simulink model "PMSG"  (Simulink 8.1)
settings: Solver=ode45  StartTime=0.0  StopTime=10  RelTol=1e-3
libraries: simulink x1
settings Model: Creator=korichi  LastModifiedBy=apple
settings SolverCC: ZeroCrossAlgorithm=Adaptive
settings OptimizationCC: InitFltsAndDblsToZero=on
settings DebuggingCC: StrictBusMsg=Warning

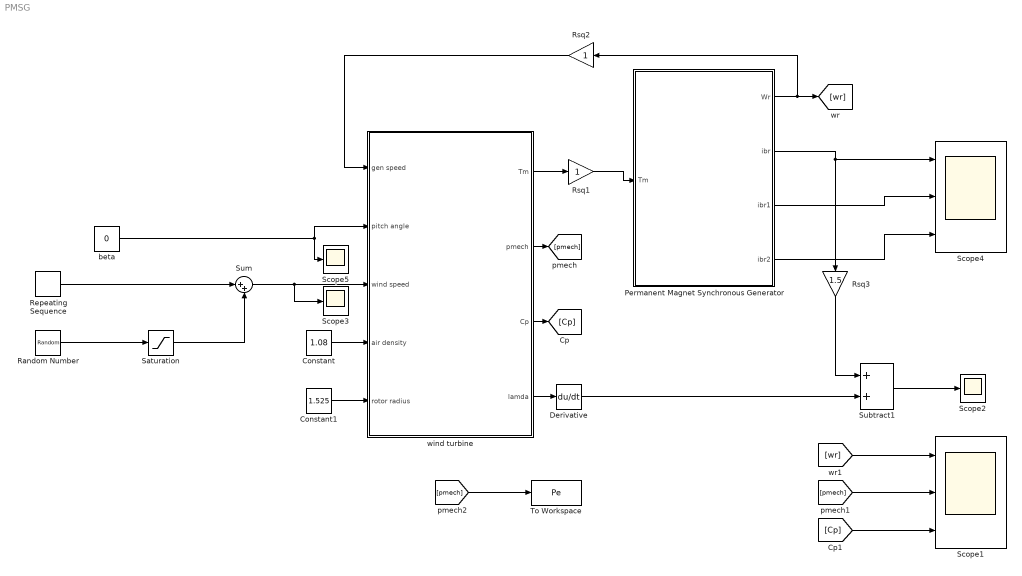
== system PMSG ==
  Constant : Constant  Value=1.08
  Constant1 : Constant  Value=1.525
  Derivative : Derivative
  Permanent Magnet Synchronous Generator : Subsystem
  Random Number : RandomNumber  Seed=20  SampleTime=0
  Repeating Sequence : simulink/Sources/Repeating Sequence  rep_seq_t=[0 2]  rep_seq_y=[0 2]
  Rsq1 : Gain
  Rsq2 : Gain
  Rsq3 : Gain  Gain=1.5
  Saturation : Saturate  UpperLimit=12  LowerLimit=5
  Scope1 : Scope  NumInputPorts=3
      settings: YMin=200~0~-0.3  YMax=650~10000~0.3  SaveName=TeW2  MaxDataPoints=100000000
  Scope2 : Scope
      settings: TimeRange=10  YMin=-9  YMax=9  SaveName=TeW  MaxDataPoints=100000000  SampleInput=on
  Scope3 : Scope
      settings: TimeRange=10  YMin=5  YMax=20  SaveName=TeW3  MaxDataPoints=100000000  SampleInput=on
  Scope4 : Scope  NumInputPorts=3
      settings: YMin=-0.7~-0.7~-0.7  YMax=0.7~0.7~0.7  SaveName=TeW1  MaxDataPoints=100000000
  Scope5 : Scope
      settings: TimeRange=10  YMin=0  YMax=55  SaveName=TeW4  MaxDataPoints=100000000  SampleInput=on
  Subtract1 : Sum
  Sum : Sum  Inputs=|++
  To Workspace : ToWorkspace  VariableName=Pe  SampleTime=-1  SaveFormat=Structure
  beta : Constant  Value=0
  wind turbine : Subsystem
  wires:
  Constant/1 -> wind turbine/4(air density)
  Constant1/1 -> wind turbine/5(rotor radius)
  wind turbine/1(Tm) -> Rsq1/1
  Sum/1 -> wind turbine/3(wind speed), Scope3/1
  Rsq2/1 -> wind turbine/1(gen speed)
  Rsq1/1 -> Permanent Magnet Synchronous Generator/1(Tm)
  wind turbine/3(Cp) -> [Cp]
  wind turbine/2(pmech) -> [pmech]
  [Cp] -> Scope1/3
  [pmech] -> Scope1/2
  [wr] -> Scope1/1
  Permanent Magnet Synchronous Generator/2(ibr) -> Scope4/1, Rsq3/1
  Rsq3/1 -> Subtract1/1
  wind turbine/4(lamda) -> Derivative/1
  Derivative/1 -> Subtract1/2
  Permanent Magnet Synchronous Generator/1(Wr) -> Rsq2/1, [wr]
  Saturation/1 -> Sum/2
  Subtract1/1 -> Scope2/1
  [pmech] -> To Workspace/1
  Permanent Magnet Synchronous Generator/3(ibr1) -> Scope4/2
  Permanent Magnet Synchronous Generator/4(ibr2) -> Scope4/3
  beta/1 -> wind turbine/2(pitch angle), Scope5/1
  Random Number/1 -> Saturation/1
  Repeating Sequence/1 -> Sum/1

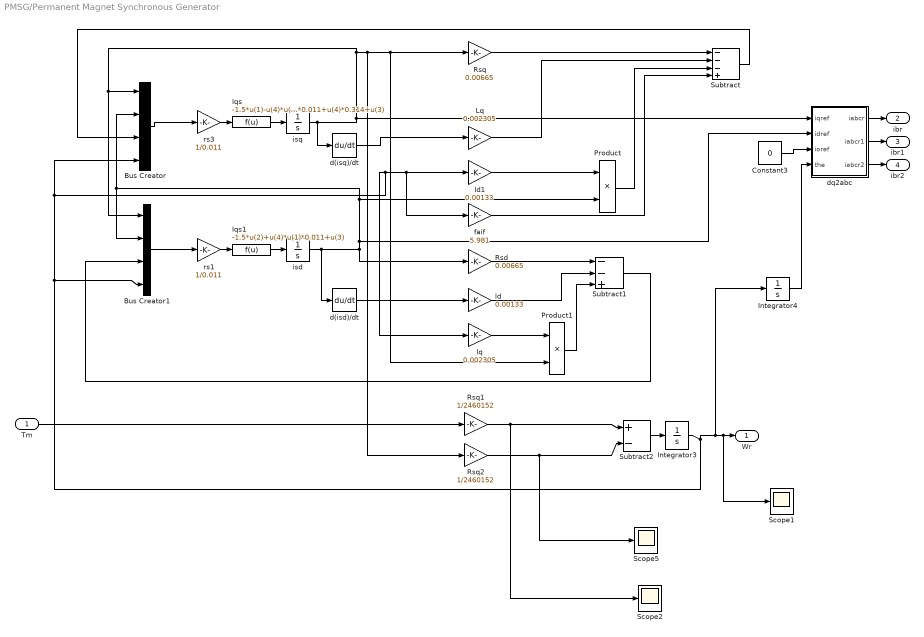
== system PMSG/Permanent Magnet Synchronous Generator ==
  Tm : Inport
  Bus Creator : BusCreator
  Bus Creator1 : BusCreator
  Constant3 : Constant  Value=0
  Integrator3 : Integrator  InitialCondition=1  IgnoreLimit=on
  Integrator4 : Integrator
  Iqs : Fcn  Expr=-1.5*u(1)-u(4)*u(2)*0.011+u(4)*0.314+u(3)
  Iqs1 : Fcn  Expr=-1.5*u(2)+u(4)*u(1)*0.011+u(3)
  Lq : Gain  Gain=0.002305
  Product : Product  RndMeth=Zero
  Product1 : Product  RndMeth=Zero
  Rsd : Gain  Gain=0.00665
  Rsq : Gain  Gain=0.00665  SampleTime=0.00665
  Rsq1 : Gain  Gain=1/2460152
  Rsq2 : Gain  Gain=1/2460152
  Scope1 : Scope
      settings: TimeRange=10  YMin=150  YMax=425  SaveName=TeW6  MaxDataPoints=100000000  SampleInput=on
  Scope2 : Scope
      settings: TimeRange=10  YMin=46.6  YMax=48.3  SaveName=TeW7  MaxDataPoints=100000000  SampleInput=on
  Scope5 : Scope
      settings: TimeRange=10  YMin=0.0035  YMax=0.00625  SaveName=TeW5  MaxDataPoints=100000000  SampleInput=on
  Subtract : Sum  Inputs=---+
  Subtract1 : Sum  Inputs=--+
  Subtract2 : Sum  Inputs=+-
  d(isd)/dt : Derivative
  d(isq)/dt : Derivative
  dq2abc : Subsystem
  faif : Gain  Gain=5.981
  isd : Integrator
  isq : Integrator
  ld : Gain  Gain=0.00133
  ld1 : Gain  Gain=0.00133
  lq : Gain  Gain=0.002305
  rs1 : Gain  Gain=1/0.011
  rs3 : Gain  Gain=1/0.011
  Wr : Outport
  ibr : Outport  Port=2
  ibr1 : Outport  Port=3
  ibr2 : Outport  Port=4
  wires:
  Rsq/1 -> Subtract/1
  Iqs/1 -> isq/1
  rs3/1 -> Iqs/1
  Bus Creator/1 -> rs3/1
  Rsq1/1 -> Scope2/1, Subtract2/1
  Rsq2/1 -> Scope5/1, Subtract2/2
  Subtract2/1 -> Integrator3/1
  Iqs1/1 -> isd/1
  rs1/1 -> Iqs1/1
  Bus Creator1/1 -> rs1/1
  Constant3/1 -> dq2abc/3(ioref)
  dq2abc/1(iabcr) -> ibr/1
  isq/1 -> Bus Creator/1, Bus Creator1/1, Rsq/1, Product1/2, Rsq2/1, dq2abc/1(iqref), d(isq)/dt/1
  isd/1 -> Bus Creator1/2, Bus Creator/2, Product/2, dq2abc/2(idref), Rsd/1, d(isd)/dt/1
  Lq/1 -> Subtract/2
  ld1/1 -> Product/1
  Product/1 -> Subtract/3
  faif/1 -> Subtract/4
  Rsd/1 -> Subtract1/1
  ld/1 -> Subtract1/2
  Subtract/1 -> Bus Creator/3
  lq/1 -> Product1/1
  Product1/1 -> Subtract1/3
  Subtract1/1 -> Bus Creator1/3
  Tm/1 -> Rsq1/1
  Integrator3/1 -> Bus Creator1/4, Bus Creator/4, lq/1, ld1/1, faif/1, Scope1/1, Wr/1, Integrator4/1
  d(isq)/dt/1 -> Lq/1
  d(isd)/dt/1 -> ld/1
  Integrator4/1 -> dq2abc/4(the)
  dq2abc/2(iabcr1) -> ibr1/1
  dq2abc/3(iabcr2) -> ibr2/1

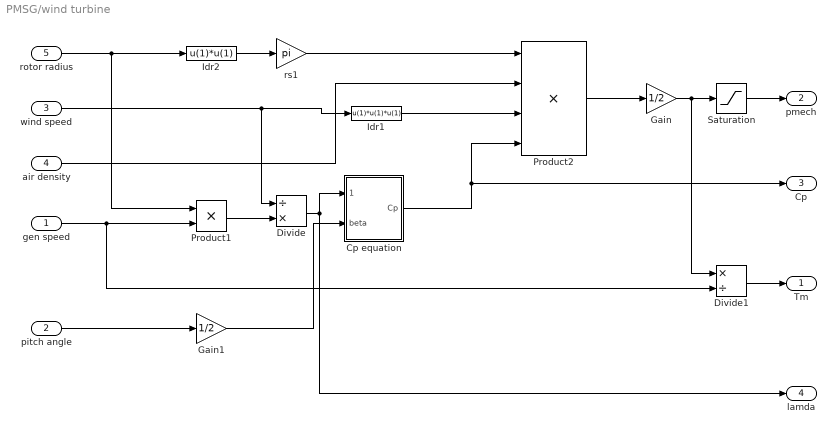
== system PMSG/wind turbine ==
  gen speed : Inport
  pitch angle : Inport  Port=2
  wind speed : Inport  Port=3
  air density : Inport  Port=4
  rotor radius : Inport  Port=5
  Cp equation : Subsystem
  Divide : Product  Inputs=/*
  Divide1 : Product  Inputs=*/
  Gain : Gain  Gain=1/2
  Gain1 : Gain  Gain=1/2
  Idr1 : Fcn  Expr=u(1)*u(1)*u(1)
  Idr2 : Fcn  Expr=u(1)*u(1)
  Product1 : Product  RndMeth=Zero
  Product2 : Product  Inputs=4  RndMeth=Zero
  Saturation : Saturate  UpperLimit=Inf  LowerLimit=0
  rs1 : Gain  Gain=pi
  Tm : Outport
  pmech : Outport  Port=2
  Cp : Outport  Port=3
  lamda : Outport  Port=4
  wires:
  gen speed/1 -> Product1/2, Divide1/2
  air density/1 -> Product2/2
  Idr1/1 -> Product2/3
  Product2/1 -> Gain/1
  rotor radius/1 -> Product1/1, Idr2/1
  wind speed/1 -> Idr1/1, Divide/1
  Product1/1 -> Divide/2
  pitch angle/1 -> Gain1/1
  rs1/1 -> Product2/1
  Idr2/1 -> rs1/1
  Divide1/1 -> Tm/1
  Gain1/1 -> Cp equation/2(beta)
  Gain/1 -> Saturation/1, Divide1/1
  Saturation/1 -> pmech/1
  Divide/1 -> Cp equation/1(lamuda), lamda/1
  Cp equation/1(Cp) -> Cp/1, Product2/4

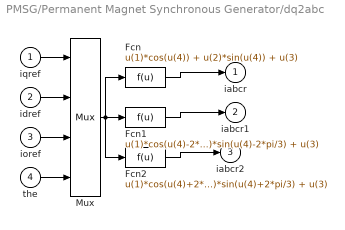
== system PMSG/Permanent Magnet Synchronous Generator/dq2abc ==
  iqref : Inport
  idref : Inport  Port=2
  ioref : Inport  Port=3
  the : Inport  Port=4
  Fcn : Fcn  Expr=u(1)*cos(u(4)) + u(2)*sin(u(4)) + u(3)
  Fcn1 : Fcn  Expr=u(1)*cos(u(4)-2*pi/3) + u(2)*sin(u(4)-2*pi/3) + u(3)
  Fcn2 : Fcn  Expr=u(1)*cos(u(4)+2*pi/3) + u(2)*sin(u(4)+2*pi/3) + u(3)
  Mux : Mux
  iabcr : Outport  InitialOutput=0
  iabcr1 : Outport  Port=2  InitialOutput=0
  iabcr2 : Outport  Port=3  InitialOutput=0
  wires:
  the/1 -> Mux/4
  ioref/1 -> Mux/3
  idref/1 -> Mux/2
  iqref/1 -> Mux/1
  Mux/1 -> Fcn1/1, Fcn2/1, Fcn/1
  Fcn1/1 -> iabcr1/1
  Fcn/1 -> iabcr/1
  Fcn2/1 -> iabcr2/1

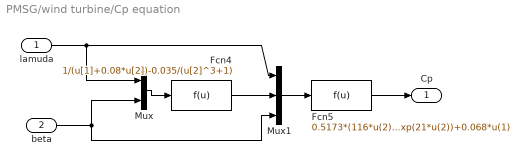
== system PMSG/wind turbine/Cp equation ==
  lamuda : Inport
  beta : Inport  Port=2
  Fcn4 : Fcn  Expr=1/(u[1]+0.08*u[2])-0.035/(u[2]^3+1)
  Fcn5 : Fcn  Expr=0.5173*(116*u(2)-0.4*u(3)-5)*exp(21*u(2))+0.068*u(1)
  Mux : Mux  Inputs=2
  Mux1 : Mux  Inputs=3
  Cp : Outport
  wires:
  beta/1 -> Mux/2, Mux1/3
  lamuda/1 -> Mux1/1, Mux/1
  Mux/1 -> Fcn4/1
  Fcn4/1 -> Mux1/2
  Mux1/1 -> Fcn5/1
  Fcn5/1 -> Cp/1
